simulink model "sim_BTMS"  (R2022b)
settings: Solver=FixedStepAuto  StartTime=0.0  StopTime=SimPara.t_sim  FixedStep=0.001  RelTol=1e-3
values from neighbouring files (symbols this model uses):
  BatPara = get_BatPara(BatPara, config_battery)    [sim_BTMS_interface.m]
  p = epe_mod(jj).p    [main_sim_BTMS_1_system_setup.m]
  SysPara = rmfield(SysPara, {'p','s'})    [main_sim_BTMS_1_system_setup.m]
undefined symbols (not defined in the file or in its folder): A, BTMSConfig, i, LSAPara, SimPara, x2_cal, x3_cal, x_cal
libraries: simulink x14, dspstat3 x7, dspindex x1
(part 4 of 4)

== system sim_BTMS/Monitoring and Logging/Load Spectrum Analysis/Load Spectrum Analysis ON/Load Spectrum Analysis ON/One parametric LSA of cell delta C-Rate/For Iterator val1 ==
  data_in : Inport
  data_in_delay : Inport  Port=2
  Add : Sum
  Assignment Subsystem : Subsystem  TreatAsAtomicUnit=on
  Constant : Constant  Value=bins_borders
  Constant2 : Constant
  Find Nonzero Elements : Find
  Iterate number of bins : ForIterator  ResetStates=reset  IterationLimit=length(bins_mean)  IterationVariableDataType=double
  Logical Operator : Logic  AllPortsSameDT=off  OutDataTypeStr=boolean
  Relational Operator : RelationalOperator  OutDataTypeStr=boolean  RndMeth=Simplest  InputSameDT=off
  Relational Operator1 : RelationalOperator  Operator=<  OutDataTypeStr=boolean  RndMeth=Simplest  InputSameDT=off
  select bin upper border : Selector  InputPortWidth=length(bins_borders)  IndexOptions=Index vector (port)  Indices=1:p  OutputSizes=1
  select parallel cell2 : Selector  InputPortWidth=length(bins_borders)  IndexOptions=Index vector (port)  Indices=1:p  OutputSizes=1
  LSA_out : Outport  VectorParamsAs1DForOutWhenUnconnected=off
  wires:
  data_in_delay/1 -> Assignment Subsystem/3(data_in_delayed)
  Constant/1 -> select bin upper border/1, select parallel cell2/1
  Add/1 -> select bin upper border/2
  Constant2/1 -> Add/1
  Iterate number of bins/1 -> Add/2, Assignment Subsystem/1(k), select parallel cell2/2
  select parallel cell2/1 -> Relational Operator/2
  select bin upper border/1 -> Relational Operator1/2
  data_in/1 -> Relational Operator1/1, Relational Operator/1
  Relational Operator1/1 -> Logical Operator/2
  Relational Operator/1 -> Logical Operator/1
  Logical Operator/1 -> Find Nonzero Elements/1
  Find Nonzero Elements/1 -> Assignment Subsystem/2(index_cell)
  Assignment Subsystem/1(LSA_out) -> LSA_out/1

== system sim_BTMS/Monitoring and Logging/Load Spectrum Analysis/Load Spectrum Analysis ON/Load Spectrum Analysis ON/One parametric LSA of cell delta temperature/For Iterator val1 ==
  data_in : Inport
  data_in_delay : Inport  Port=2
  Add : Sum
  Assignment Subsystem : Subsystem  TreatAsAtomicUnit=on
  Constant : Constant  Value=bins_borders
  Constant2 : Constant
  Find Nonzero Elements : Find
  Iterate number of bins : ForIterator  ResetStates=reset  IterationLimit=length(bins_mean)  IterationVariableDataType=double
  Logical Operator : Logic  AllPortsSameDT=off  OutDataTypeStr=boolean
  Relational Operator : RelationalOperator  OutDataTypeStr=boolean  RndMeth=Simplest  InputSameDT=off
  Relational Operator1 : RelationalOperator  Operator=<  OutDataTypeStr=boolean  RndMeth=Simplest  InputSameDT=off
  select bin upper border : Selector  InputPortWidth=length(bins_borders)  IndexOptions=Index vector (port)  Indices=1:p  OutputSizes=1
  select parallel cell2 : Selector  InputPortWidth=length(bins_borders)  IndexOptions=Index vector (port)  Indices=1:p  OutputSizes=1
  LSA_out : Outport  VectorParamsAs1DForOutWhenUnconnected=off
  wires:
  Assignment Subsystem/1(LSA_out) -> LSA_out/1
  Find Nonzero Elements/1 -> Assignment Subsystem/2(index_cell)
  Logical Operator/1 -> Find Nonzero Elements/1
  Relational Operator/1 -> Logical Operator/1
  Relational Operator1/1 -> Logical Operator/2
  data_in/1 -> Relational Operator/1, Relational Operator1/1
  select bin upper border/1 -> Relational Operator1/2
  select parallel cell2/1 -> Relational Operator/2
  Iterate number of bins/1 -> select parallel cell2/2, Assignment Subsystem/1(k), Add/2
  Constant2/1 -> Add/1
  Add/1 -> select bin upper border/2
  Constant/1 -> select parallel cell2/1, select bin upper border/1
  data_in_delay/1 -> Assignment Subsystem/3(data_in_delayed)

== system sim_BTMS/Monitoring and Logging/Load Spectrum Analysis/Load Spectrum Analysis ON/Load Spectrum Analysis ON/One parametric LSA of cell temperatures/For Iterator val1 ==
  data_in : Inport
  data_in_delay : Inport  Port=2
  Add : Sum
  Assignment Subsystem : Subsystem  TreatAsAtomicUnit=on
  Constant : Constant  Value=bins_borders
  Constant2 : Constant
  Find Nonzero Elements : Find
  Iterate number of bins : ForIterator  ResetStates=reset  IterationLimit=length(bins_mean)  IterationVariableDataType=double
  Logical Operator : Logic  AllPortsSameDT=off  OutDataTypeStr=boolean
  Relational Operator : RelationalOperator  OutDataTypeStr=boolean  RndMeth=Simplest  InputSameDT=off
  Relational Operator1 : RelationalOperator  Operator=<  OutDataTypeStr=boolean  RndMeth=Simplest  InputSameDT=off
  select bin upper border : Selector  InputPortWidth=length(bins_borders)  IndexOptions=Index vector (port)  Indices=1:p  OutputSizes=1
  select parallel cell2 : Selector  InputPortWidth=length(bins_borders)  IndexOptions=Index vector (port)  Indices=1:p  OutputSizes=1
  LSA_out : Outport  VectorParamsAs1DForOutWhenUnconnected=off
  wires:
  Assignment Subsystem/1(LSA_out) -> LSA_out/1
  Find Nonzero Elements/1 -> Assignment Subsystem/2(index_cell)
  Logical Operator/1 -> Find Nonzero Elements/1
  Relational Operator/1 -> Logical Operator/1
  Relational Operator1/1 -> Logical Operator/2
  data_in/1 -> Relational Operator/1, Relational Operator1/1
  select bin upper border/1 -> Relational Operator1/2
  select parallel cell2/1 -> Relational Operator/2
  Iterate number of bins/1 -> select parallel cell2/2, Assignment Subsystem/1(k), Add/2
  Constant2/1 -> Add/1
  Add/1 -> select bin upper border/2
  Constant/1 -> select parallel cell2/1, select bin upper border/1
  data_in_delay/1 -> Assignment Subsystem/3(data_in_delayed)

== system sim_BTMS/Monitoring and Logging/Load Spectrum Analysis/Load Spectrum Analysis ON/Load Spectrum Analysis ON/Subsystem1/SubsyMMatrssdatrixm ==
  In1 : Inport
  Enable : EnablePort  PropagateVarSize=During execution
  "summiert Dim. 4, die die Einzelzelle angibt" : Sum  Inputs=+  CollapseMode=Specified dimension  CollapseDim=dim
  Out1 : Outport  VectorParamsAs1DForOutWhenUnconnected=off
  wires:
  In1/1 -> "summiert Dim. 4, die die Einzelzelle angibt"/1
  "summiert Dim. 4, die die Einzelzelle angibt"/1 -> Out1/1

== system sim_BTMS/Monitoring and Logging/Load Spectrum Analysis/Load Spectrum Analysis ON/Load Spectrum Analysis ON/Subsystem2/SubsyMMatrssdatrixm ==
  In1 : Inport
  Enable : EnablePort  PropagateVarSize=During execution
  "summiert Dim. 4, die die Einzelzelle angibt" : Sum  Inputs=+  CollapseMode=Specified dimension  CollapseDim=dim
  Out1 : Outport  VectorParamsAs1DForOutWhenUnconnected=off
  wires:
  "summiert Dim. 4, die die Einzelzelle angibt"/1 -> Out1/1
  In1/1 -> "summiert Dim. 4, die die Einzelzelle angibt"/1

== system sim_BTMS/Monitoring and Logging/Load Spectrum Analysis/Load Spectrum Analysis ON/Load Spectrum Analysis ON/Subsystem3/SubsyMMatrssdatrixm ==
  In1 : Inport
  Enable : EnablePort  PropagateVarSize=During execution
  "summiert Dim. 4, die die Einzelzelle angibt" : Sum  Inputs=+  CollapseMode=Specified dimension  CollapseDim=dim
  Out1 : Outport  VectorParamsAs1DForOutWhenUnconnected=off
  wires:
  In1/1 -> "summiert Dim. 4, die die Einzelzelle angibt"/1
  "summiert Dim. 4, die die Einzelzelle angibt"/1 -> Out1/1

== system sim_BTMS/Monitoring and Logging/Load Spectrum Analysis/Load Spectrum Analysis ON/Load Spectrum Analysis ON/Subsystem4/SubsyMMatrssdatrixm ==
  In1 : Inport
  Enable : EnablePort  PropagateVarSize=During execution
  "summiert Dim. 4, die die Einzelzelle angibt" : Sum  Inputs=+  CollapseMode=Specified dimension  CollapseDim=dim
  Out1 : Outport  VectorParamsAs1DForOutWhenUnconnected=off
  wires:
  "summiert Dim. 4, die die Einzelzelle angibt"/1 -> Out1/1
  In1/1 -> "summiert Dim. 4, die die Einzelzelle angibt"/1

== system sim_BTMS/Monitoring and Logging/Load Spectrum Analysis/Load Spectrum Analysis ON/Load Spectrum Analysis ON/Subsystem5/SubsyMMatrssdatrixm ==
  In1 : Inport
  Enable : EnablePort  PropagateVarSize=During execution
  "summiert Dim. 4, die die Einzelzelle angibt" : Sum  Inputs=+  CollapseMode=Specified dimension  CollapseDim=dim
  Out1 : Outport  VectorParamsAs1DForOutWhenUnconnected=off
  wires:
  In1/1 -> "summiert Dim. 4, die die Einzelzelle angibt"/1
  "summiert Dim. 4, die die Einzelzelle angibt"/1 -> Out1/1

== system sim_BTMS/Monitoring and Logging/Load Spectrum Analysis/Load Spectrum Analysis ON/Load Spectrum Analysis ON/Subsystem6/SubsyMMatrssdatrixm ==
  In1 : Inport
  Enable : EnablePort  PropagateVarSize=During execution
  "summiert Dim. 4, die die Einzelzelle angibt" : Sum  Inputs=+  CollapseMode=Specified dimension  CollapseDim=dim
  Out1 : Outport  VectorParamsAs1DForOutWhenUnconnected=off
  wires:
  "summiert Dim. 4, die die Einzelzelle angibt"/1 -> Out1/1
  In1/1 -> "summiert Dim. 4, die die Einzelzelle angibt"/1

== system sim_BTMS/Monitoring and Logging/Load Spectrum Analysis/Load Spectrum Analysis ON/Load Spectrum Analysis ON/Subsystem7/SubsyMMatrssdatrixm ==
  In1 : Inport
  Enable : EnablePort  PropagateVarSize=During execution
  "summiert Dim. 4, die die Einzelzelle angibt" : Sum  Inputs=+  CollapseMode=Specified dimension  CollapseDim=dim
  Out1 : Outport  VectorParamsAs1DForOutWhenUnconnected=off
  wires:
  In1/1 -> "summiert Dim. 4, die die Einzelzelle angibt"/1
  "summiert Dim. 4, die die Einzelzelle angibt"/1 -> Out1/1

== system sim_BTMS/Monitoring and Logging/Load Spectrum Analysis/Load Spectrum Analysis ON/Load Spectrum Analysis ON/Subsystem8/SubsyMMatrssdatrixm ==
  In1 : Inport
  Enable : EnablePort  PropagateVarSize=During execution
  "summiert Dim. 4, die die Einzelzelle angibt" : Sum  Inputs=+  CollapseMode=Specified dimension  CollapseDim=dim
  Out1 : Outport  VectorParamsAs1DForOutWhenUnconnected=off
  wires:
  In1/1 -> "summiert Dim. 4, die die Einzelzelle angibt"/1
  "summiert Dim. 4, die die Einzelzelle angibt"/1 -> Out1/1

== system sim_BTMS/Monitoring and Logging/Load Spectrum Analysis/Load Spectrum Analysis ON/Load Spectrum Analysis ON/Subsystem9/SubsyMMatrssdatrixm ==
  In1 : Inport
  Enable : EnablePort  PropagateVarSize=During execution
  "summiert Dim. 4, die die Einzelzelle angibt" : Sum  Inputs=+  CollapseMode=Specified dimension  CollapseDim=dim
  Out1 : Outport  VectorParamsAs1DForOutWhenUnconnected=off
  wires:
  "summiert Dim. 4, die die Einzelzelle angibt"/1 -> Out1/1
  In1/1 -> "summiert Dim. 4, die die Einzelzelle angibt"/1

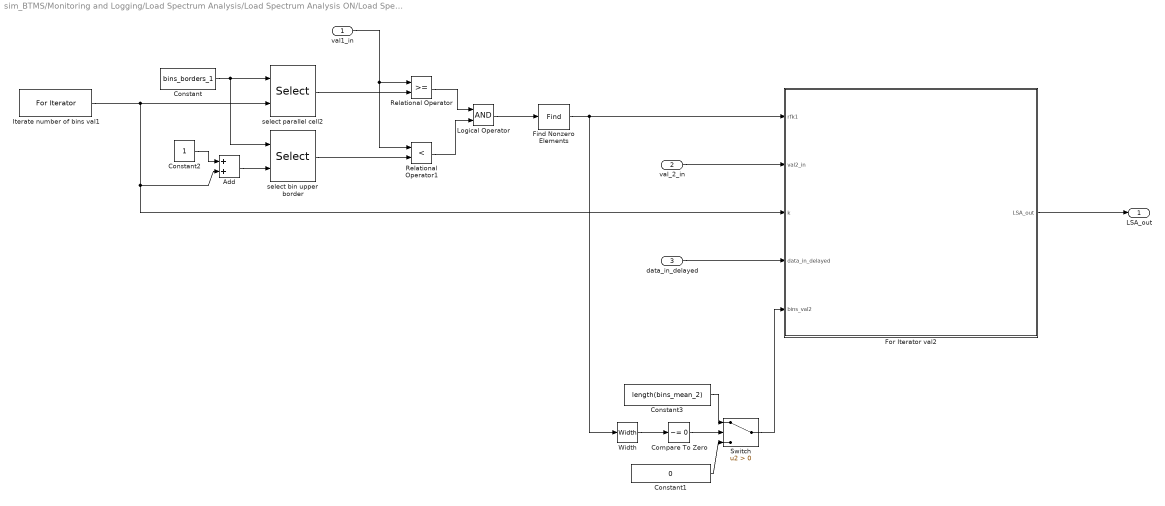
== system sim_BTMS/Monitoring and Logging/Load Spectrum Analysis/Load Spectrum Analysis ON/Load Spectrum Analysis ON/Two parametric LSA of cell C-Rate vs. temperature/For Iterator val1 ==
  val1_in : Inport
  val_2_in : Inport  Port=2
  data_in_delayed : Inport  Port=3
  Add : Sum
  Compare To Zero : simulink/Logic and Bit Operations/Compare To Zero  relop=~=  OutDataTypeStr=boolean
  Constant : Constant  Value=bins_borders_1
  Constant1 : Constant  Value=0
  Constant2 : Constant
  Constant3 : Constant  Value=length(bins_mean_2)
  Find Nonzero Elements : Find
  "For Iterator val2 " : Subsystem  TreatAsAtomicUnit=on
  Iterate number of bins val1 : ForIterator  ResetStates=reset  IterationLimit=length(bins_mean_1)  IterationVariableDataType=double
  Logical Operator : Logic  AllPortsSameDT=off  OutDataTypeStr=boolean
  Relational Operator : RelationalOperator  OutDataTypeStr=boolean  RndMeth=Simplest  InputSameDT=off
  Relational Operator1 : RelationalOperator  Operator=<  OutDataTypeStr=boolean  RndMeth=Simplest  InputSameDT=off
  Switch : Switch  Criteria=u2 > Threshold  SaturateOnIntegerOverflow=off  InputSameDT=off
  Width : Width
  select bin upper border : Selector  InputPortWidth=length(bins_borders_1)  IndexOptions=Index vector (port)  Indices=1:p  OutputSizes=1
  select parallel cell2 : Selector  InputPortWidth=length(bins_borders_1)  IndexOptions=Index vector (port)  Indices=1:p  OutputSizes=1
  LSA_out : Outport  VectorParamsAs1DForOutWhenUnconnected=off
  wires:
  val_2_in/1 -> "For Iterator val2 "/2(val2_in)
  Find Nonzero Elements/1 -> "For Iterator val2 "/1(rfk1), Width/1
  Logical Operator/1 -> Find Nonzero Elements/1
  Relational Operator/1 -> Logical Operator/1
  Relational Operator1/1 -> Logical Operator/2
  val1_in/1 -> Relational Operator/1, Relational Operator1/1
  select bin upper border/1 -> Relational Operator1/2
  select parallel cell2/1 -> Relational Operator/2
  Iterate number of bins val1/1 -> select parallel cell2/2, Add/2, "For Iterator val2 "/3(k)
  Constant2/1 -> Add/1
  Add/1 -> select bin upper border/2
  Constant/1 -> select parallel cell2/1, select bin upper border/1
  "For Iterator val2 "/1(LSA_out) -> LSA_out/1
  data_in_delayed/1 -> "For Iterator val2 "/4(data_in_delayed)
  Compare To Zero/1 -> Switch/2
  Constant1/1 -> Switch/3
  Width/1 -> Compare To Zero/1
  Switch/1 -> "For Iterator val2 "/5(bins_val2)
  Constant3/1 -> Switch/1

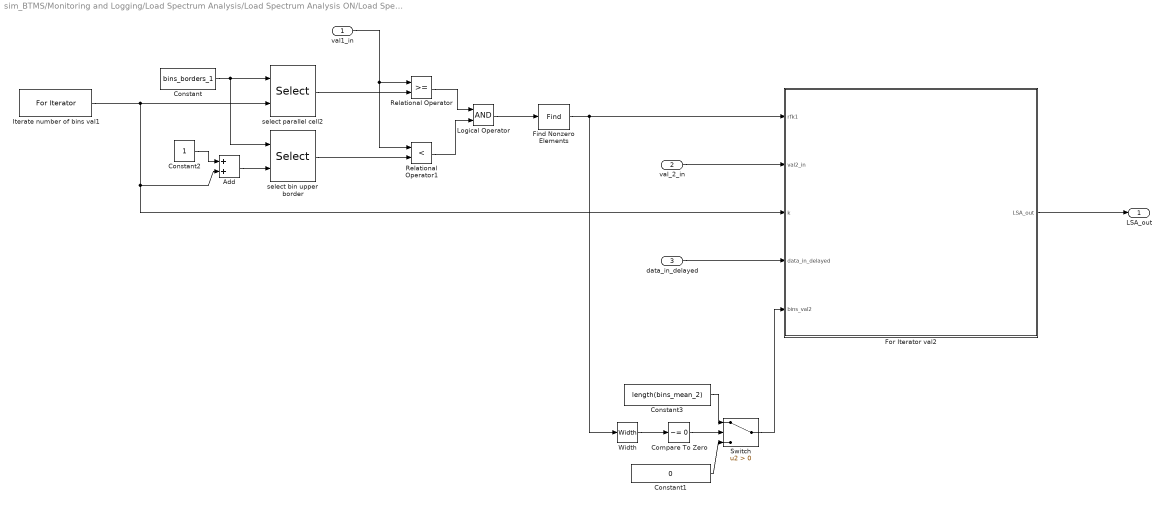
== system sim_BTMS/Monitoring and Logging/Load Spectrum Analysis/Load Spectrum Analysis ON/Load Spectrum Analysis ON/Two parametric LSA of cell SOC vs. C-Rate/For Iterator val1 ==
  val1_in : Inport
  val_2_in : Inport  Port=2
  data_in_delayed : Inport  Port=3
  Add : Sum
  Compare To Zero : simulink/Logic and Bit Operations/Compare To Zero  relop=~=  OutDataTypeStr=boolean
  Constant : Constant  Value=bins_borders_1
  Constant1 : Constant  Value=0
  Constant2 : Constant
  Constant3 : Constant  Value=length(bins_mean_2)
  Find Nonzero Elements : Find
  "For Iterator val2 " : Subsystem  TreatAsAtomicUnit=on
  Iterate number of bins val1 : ForIterator  ResetStates=reset  IterationLimit=length(bins_mean_1)  IterationVariableDataType=double
  Logical Operator : Logic  AllPortsSameDT=off  OutDataTypeStr=boolean
  Relational Operator : RelationalOperator  OutDataTypeStr=boolean  RndMeth=Simplest  InputSameDT=off
  Relational Operator1 : RelationalOperator  Operator=<  OutDataTypeStr=boolean  RndMeth=Simplest  InputSameDT=off
  Switch : Switch  Criteria=u2 > Threshold  SaturateOnIntegerOverflow=off  InputSameDT=off
  Width : Width
  select bin upper border : Selector  InputPortWidth=length(bins_borders_1)  IndexOptions=Index vector (port)  Indices=1:p  OutputSizes=1
  select parallel cell2 : Selector  InputPortWidth=length(bins_borders_1)  IndexOptions=Index vector (port)  Indices=1:p  OutputSizes=1
  LSA_out : Outport  VectorParamsAs1DForOutWhenUnconnected=off
  wires:
  Constant3/1 -> Switch/1
  Switch/1 -> "For Iterator val2 "/5(bins_val2)
  Width/1 -> Compare To Zero/1
  Constant1/1 -> Switch/3
  Compare To Zero/1 -> Switch/2
  data_in_delayed/1 -> "For Iterator val2 "/4(data_in_delayed)
  "For Iterator val2 "/1(LSA_out) -> LSA_out/1
  Constant/1 -> select bin upper border/1, select parallel cell2/1
  Add/1 -> select bin upper border/2
  Constant2/1 -> Add/1
  Iterate number of bins val1/1 -> "For Iterator val2 "/3(k), Add/2, select parallel cell2/2
  select parallel cell2/1 -> Relational Operator/2
  select bin upper border/1 -> Relational Operator1/2
  val1_in/1 -> Relational Operator1/1, Relational Operator/1
  Relational Operator1/1 -> Logical Operator/2
  Relational Operator/1 -> Logical Operator/1
  Logical Operator/1 -> Find Nonzero Elements/1
  Find Nonzero Elements/1 -> Width/1, "For Iterator val2 "/1(rfk1)
  val_2_in/1 -> "For Iterator val2 "/2(val2_in)

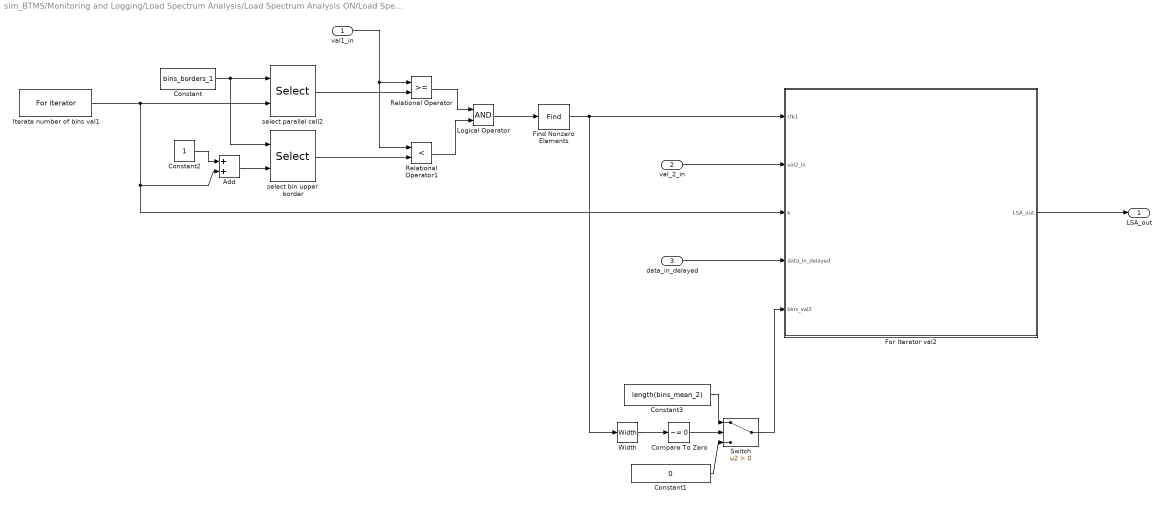
== system sim_BTMS/Monitoring and Logging/Load Spectrum Analysis/Load Spectrum Analysis ON/Load Spectrum Analysis ON/Two parametric LSA of cell SOC vs. temperature /For Iterator val1 ==
  val1_in : Inport
  val_2_in : Inport  Port=2
  data_in_delayed : Inport  Port=3
  Add : Sum
  Compare To Zero : simulink/Logic and Bit Operations/Compare To Zero  relop=~=  OutDataTypeStr=boolean
  Constant : Constant  Value=bins_borders_1
  Constant1 : Constant  Value=0
  Constant2 : Constant
  Constant3 : Constant  Value=length(bins_mean_2)
  Find Nonzero Elements : Find
  "For Iterator val2 " : Subsystem  TreatAsAtomicUnit=on
  Iterate number of bins val1 : ForIterator  ResetStates=reset  IterationLimit=length(bins_mean_1)  IterationVariableDataType=double
  Logical Operator : Logic  AllPortsSameDT=off  OutDataTypeStr=boolean
  Relational Operator : RelationalOperator  OutDataTypeStr=boolean  RndMeth=Simplest  InputSameDT=off
  Relational Operator1 : RelationalOperator  Operator=<  OutDataTypeStr=boolean  RndMeth=Simplest  InputSameDT=off
  Switch : Switch  Criteria=u2 > Threshold  SaturateOnIntegerOverflow=off  InputSameDT=off
  Width : Width
  select bin upper border : Selector  InputPortWidth=length(bins_borders_1)  IndexOptions=Index vector (port)  Indices=1:p  OutputSizes=1
  select parallel cell2 : Selector  InputPortWidth=length(bins_borders_1)  IndexOptions=Index vector (port)  Indices=1:p  OutputSizes=1
  LSA_out : Outport  VectorParamsAs1DForOutWhenUnconnected=off
  wires:
  Constant3/1 -> Switch/1
  Switch/1 -> "For Iterator val2 "/5(bins_val2)
  Width/1 -> Compare To Zero/1
  Constant1/1 -> Switch/3
  Compare To Zero/1 -> Switch/2
  data_in_delayed/1 -> "For Iterator val2 "/4(data_in_delayed)
  "For Iterator val2 "/1(LSA_out) -> LSA_out/1
  Constant/1 -> select bin upper border/1, select parallel cell2/1
  Add/1 -> select bin upper border/2
  Constant2/1 -> Add/1
  Iterate number of bins val1/1 -> "For Iterator val2 "/3(k), Add/2, select parallel cell2/2
  select parallel cell2/1 -> Relational Operator/2
  select bin upper border/1 -> Relational Operator1/2
  val1_in/1 -> Relational Operator1/1, Relational Operator/1
  Relational Operator1/1 -> Logical Operator/2
  Relational Operator/1 -> Logical Operator/1
  Logical Operator/1 -> Find Nonzero Elements/1
  Find Nonzero Elements/1 -> Width/1, "For Iterator val2 "/1(rfk1)
  val_2_in/1 -> "For Iterator val2 "/2(val2_in)

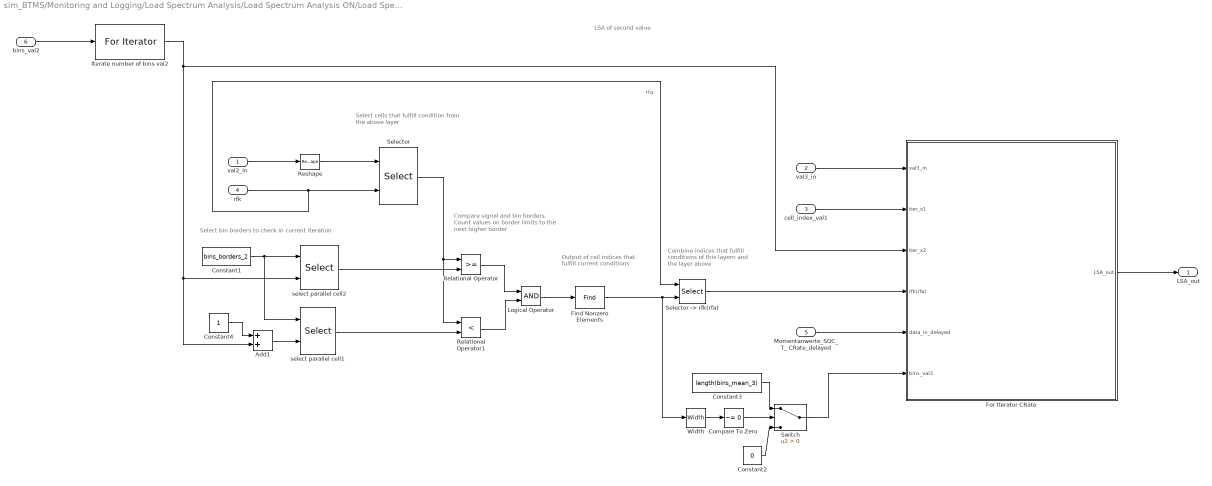
== system sim_BTMS/Monitoring and Logging/Load Spectrum Analysis/Load Spectrum Analysis ON/Load Spectrum Analysis ON/3-parametrische Momentanwertzählung SOC, T_Cells, CRate/For Iterator val1/For Iterator val2 ==
  note: Select cells that fulfill condition from the above layer
  note: LSA of second value
  note: rfa
  note: Select bin borders to check in current iteration
  note: Compare signal and bin borders. Count values on border limits to the next higher border
  note: Output of cell indices that fulfill current conditions
  note: Combine indices that fulfill conditions of this layern and the layer above
  val2_in : Inport
  val3_in : Inport  Port=2
  cell_index_val1 : Inport  Port=3
  rfk : Inport  Port=4
  Momentanwerte_SOC_T_ CRate_delayed : Inport  Port=5
  bins_val2 : Inport  Port=6
  Add1 : Sum
  Compare To Zero : simulink/Logic and Bit Operations/Compare To Zero  relop=~=  OutDataTypeStr=boolean
  Constant1 : Constant  Value=bins_borders_2
  Constant2 : Constant  Value=0
  Constant3 : Constant  Value=length(bins_mean_3)
  Constant4 : Constant
  Find Nonzero Elements : Find
  For Iterator CRate : Subsystem  TreatAsAtomicUnit=on
  Iterate number of bins val2 : ForIterator  ResetStates=reset  IterationSource=external  IterationLimit=length(x2_cal)  IterationVariableDataType=double
  Logical Operator : Logic  AllPortsSameDT=off  OutDataTypeStr=boolean
  Relational Operator : RelationalOperator  OutDataTypeStr=boolean  RndMeth=Simplest  InputSameDT=off
  Relational Operator1 : RelationalOperator  Operator=<  OutDataTypeStr=boolean  RndMeth=Simplest  InputSameDT=off
  Reshape : Reshape
  Selector : Selector  InputPortWidth=SysPara.p*SysPara.s  IndexOptions=Index vector (port)  Indices=1:p  OutputSizes=1
  "Selector -> rfk(rfa)" : Selector  InputPortWidth=SysPara.p*SysPara.s  IndexOptions=Index vector (port)  Indices=[1 3]  OutputSizes=1
  Switch : Switch  Criteria=u2 > Threshold  SaturateOnIntegerOverflow=off  InputSameDT=off
  Width : Width
  select parallel cell1 : Selector  InputPortWidth=length(bins_borders_2)  IndexOptions=Index vector (port)  Indices=1:p  OutputSizes=1
  select parallel cell2 : Selector  InputPortWidth=length(bins_borders_2)  IndexOptions=Index vector (port)  Indices=1:p  OutputSizes=1
  LSA_out : Outport  VectorParamsAs1DForOutWhenUnconnected=off
  wires:
  Switch/1 -> For Iterator CRate/6(bins_val3)
  Constant3/1 -> Switch/1
  Width/1 -> Compare To Zero/1
  Constant2/1 -> Switch/3
  Compare To Zero/1 -> Switch/2
  Find Nonzero Elements/1 -> "Selector -> rfk(rfa)"/2, Width/1
  bins_val2/1 -> Iterate number of bins val2/1
  val3_in/1 -> For Iterator CRate/1(val3_in)
  For Iterator CRate/1(LSA_out) -> LSA_out/1
  "Selector -> rfk(rfa)"/1 -> For Iterator CRate/4(rfk(rfa))
  rfk/1 -> Selector/2, "Selector -> rfk(rfa)"/1
  Logical Operator/1 -> Find Nonzero Elements/1
  Reshape/1 -> Selector/1
  val2_in/1 -> Reshape/1
  cell_index_val1/1 -> For Iterator CRate/2(iter_x1)
  Selector/1 -> Relational Operator/1, Relational Operator1/1
  Relational Operator/1 -> Logical Operator/1
  Relational Operator1/1 -> Logical Operator/2
  select parallel cell1/1 -> Relational Operator1/2
  select parallel cell2/1 -> Relational Operator/2
  Constant4/1 -> Add1/1
  Add1/1 -> select parallel cell1/2
  Iterate number of bins val2/1 -> select parallel cell2/2, Add1/2, For Iterator CRate/3(iter_x2)
  Constant1/1 -> select parallel cell2/1, select parallel cell1/1
  Momentanwerte_SOC_T_ CRate_delayed/1 -> For Iterator CRate/5(data_in_delayed)

== system sim_BTMS/Monitoring and Logging/Load Spectrum Analysis/Load Spectrum Analysis ON/Load Spectrum Analysis ON/One parametric LSA of cell C-Rate/For Iterator val1/Assignment Subsystem ==
  k : Inport
  index_cell : Inport  Port=2
  data_in_delayed : Inport  Port=3
  Add : Sum
  Assignment of matrix entries : Assignment  NumberOfDimensions=2  OutputInitialize=Specify size for each dimension in table  IndexOptions=Index vector (port),Index vector (port)  Indices=1,1  OutputSizes=length(bins_mean),SysPara.p*SysPara.s+1
  Constant1 : Constant  Value=SimPara.t_step
  "Selection of delayed matrix entries " : Selector  NumberOfDimensions=2  InputPortWidth=3  IndexOptions=Index vector (port),Index vector (port)  Indices=[1 3],1  OutputSizes=1,1
  LSA_out : Outport  VectorParamsAs1DForOutWhenUnconnected=off
  wires:
  index_cell/1 -> Assignment of matrix entries/3, "Selection of delayed matrix entries "/3
  Assignment of matrix entries/1 -> LSA_out/1
  k/1 -> "Selection of delayed matrix entries "/2, Assignment of matrix entries/2
  Constant1/1 -> Add/1
  "Selection of delayed matrix entries "/1 -> Add/2
  Add/1 -> Assignment of matrix entries/1
  data_in_delayed/1 -> "Selection of delayed matrix entries "/1

== system sim_BTMS/Monitoring and Logging/Load Spectrum Analysis/Load Spectrum Analysis ON/Load Spectrum Analysis ON/One parametric LSA of cell SOC/For Iterator val1/Assignment Subsystem ==
  k : Inport
  index_cell : Inport  Port=2
  data_in_delayed : Inport  Port=3
  Add : Sum
  Assignment of matrix entries : Assignment  NumberOfDimensions=2  OutputInitialize=Specify size for each dimension in table  IndexOptions=Index vector (port),Index vector (port)  Indices=1,1  OutputSizes=length(bins_mean),SysPara.p*SysPara.s+1
  Constant1 : Constant  Value=SimPara.t_step
  "Selection of delayed matrix entries " : Selector  NumberOfDimensions=2  InputPortWidth=3  IndexOptions=Index vector (port),Index vector (port)  Indices=[1 3],1  OutputSizes=1,1
  LSA_out : Outport  VectorParamsAs1DForOutWhenUnconnected=off
  wires:
  data_in_delayed/1 -> "Selection of delayed matrix entries "/1
  Add/1 -> Assignment of matrix entries/1
  "Selection of delayed matrix entries "/1 -> Add/2
  Constant1/1 -> Add/1
  k/1 -> Assignment of matrix entries/2, "Selection of delayed matrix entries "/2
  Assignment of matrix entries/1 -> LSA_out/1
  index_cell/1 -> "Selection of delayed matrix entries "/3, Assignment of matrix entries/3

== system sim_BTMS/Monitoring and Logging/Load Spectrum Analysis/Load Spectrum Analysis ON/Load Spectrum Analysis ON/One parametric LSA of cell delta C-Rate/For Iterator val1/Assignment Subsystem ==
  k : Inport
  index_cell : Inport  Port=2
  data_in_delayed : Inport  Port=3
  Add : Sum
  Assignment of matrix entries : Assignment  NumberOfDimensions=2  OutputInitialize=Specify size for each dimension in table  IndexOptions=Index vector (port),Index vector (port)  Indices=1,1  OutputSizes=length(bins_mean),SysPara.p*SysPara.s+1
  Constant1 : Constant  Value=SimPara.t_step
  "Selection of delayed matrix entries " : Selector  NumberOfDimensions=2  InputPortWidth=3  IndexOptions=Index vector (port),Index vector (port)  Indices=[1 3],1  OutputSizes=1,1
  LSA_out : Outport  VectorParamsAs1DForOutWhenUnconnected=off
  wires:
  data_in_delayed/1 -> "Selection of delayed matrix entries "/1
  Add/1 -> Assignment of matrix entries/1
  "Selection of delayed matrix entries "/1 -> Add/2
  Constant1/1 -> Add/1
  k/1 -> Assignment of matrix entries/2, "Selection of delayed matrix entries "/2
  Assignment of matrix entries/1 -> LSA_out/1
  index_cell/1 -> "Selection of delayed matrix entries "/3, Assignment of matrix entries/3

== system sim_BTMS/Monitoring and Logging/Load Spectrum Analysis/Load Spectrum Analysis ON/Load Spectrum Analysis ON/One parametric LSA of cell delta temperature/For Iterator val1/Assignment Subsystem ==
  k : Inport
  index_cell : Inport  Port=2
  data_in_delayed : Inport  Port=3
  Add : Sum
  Assignment of matrix entries : Assignment  NumberOfDimensions=2  OutputInitialize=Specify size for each dimension in table  IndexOptions=Index vector (port),Index vector (port)  Indices=1,1  OutputSizes=length(bins_mean),SysPara.p*SysPara.s+1
  Constant1 : Constant  Value=SimPara.t_step
  "Selection of delayed matrix entries " : Selector  NumberOfDimensions=2  InputPortWidth=3  IndexOptions=Index vector (port),Index vector (port)  Indices=[1 3],1  OutputSizes=1,1
  LSA_out : Outport  VectorParamsAs1DForOutWhenUnconnected=off
  wires:
  index_cell/1 -> Assignment of matrix entries/3, "Selection of delayed matrix entries "/3
  Assignment of matrix entries/1 -> LSA_out/1
  k/1 -> "Selection of delayed matrix entries "/2, Assignment of matrix entries/2
  Constant1/1 -> Add/1
  "Selection of delayed matrix entries "/1 -> Add/2
  Add/1 -> Assignment of matrix entries/1
  data_in_delayed/1 -> "Selection of delayed matrix entries "/1

== system sim_BTMS/Monitoring and Logging/Load Spectrum Analysis/Load Spectrum Analysis ON/Load Spectrum Analysis ON/One parametric LSA of cell temperatures/For Iterator val1/Assignment Subsystem ==
  k : Inport
  index_cell : Inport  Port=2
  data_in_delayed : Inport  Port=3
  Add : Sum
  Assignment of matrix entries : Assignment  NumberOfDimensions=2  OutputInitialize=Specify size for each dimension in table  IndexOptions=Index vector (port),Index vector (port)  Indices=1,1  OutputSizes=length(bins_mean),SysPara.p*SysPara.s+1
  Constant1 : Constant  Value=SimPara.t_step
  "Selection of delayed matrix entries " : Selector  NumberOfDimensions=2  InputPortWidth=3  IndexOptions=Index vector (port),Index vector (port)  Indices=[1 3],1  OutputSizes=1,1
  LSA_out : Outport  VectorParamsAs1DForOutWhenUnconnected=off
  wires:
  index_cell/1 -> Assignment of matrix entries/3, "Selection of delayed matrix entries "/3
  Assignment of matrix entries/1 -> LSA_out/1
  k/1 -> "Selection of delayed matrix entries "/2, Assignment of matrix entries/2
  Constant1/1 -> Add/1
  "Selection of delayed matrix entries "/1 -> Add/2
  Add/1 -> Assignment of matrix entries/1
  data_in_delayed/1 -> "Selection of delayed matrix entries "/1

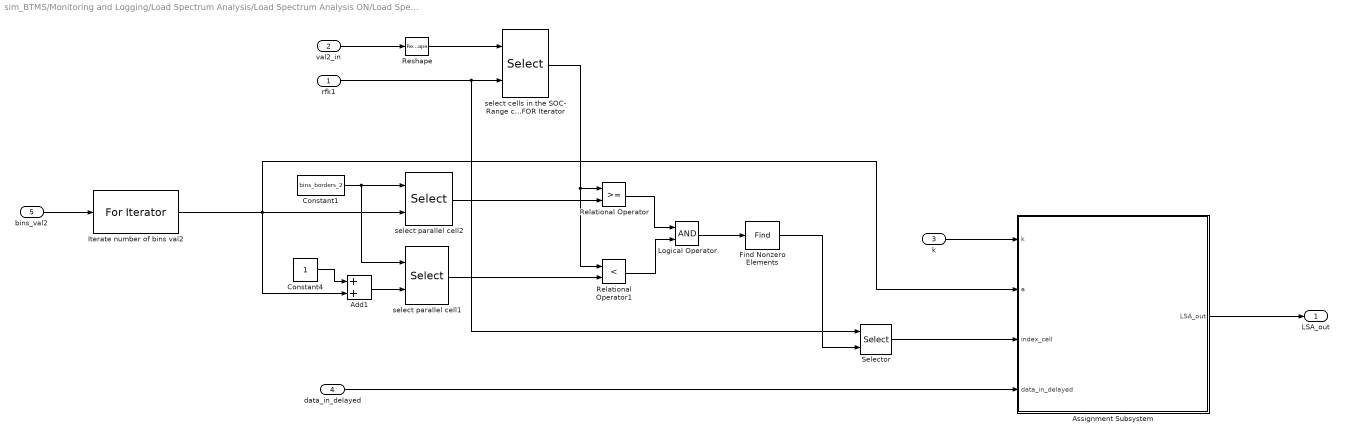
== system sim_BTMS/Monitoring and Logging/Load Spectrum Analysis/Load Spectrum Analysis ON/Load Spectrum Analysis ON/Two parametric LSA of cell C-Rate vs. temperature/For Iterator val1/For Iterator val2  ==
  rfk1 : Inport
  val2_in : Inport  Port=2
  k : Inport  Port=3
  data_in_delayed : Inport  Port=4
  bins_val2 : Inport  Port=5
  Add1 : Sum
  Assignment Subsystem : Subsystem  TreatAsAtomicUnit=on
  Constant1 : Constant  Value=bins_borders_2
  Constant4 : Constant
  Find Nonzero Elements : Find
  Iterate number of bins val2 : ForIterator  ResetStates=reset  IterationSource=external  IterationLimit=length(x_cal)  IterationVariableDataType=double
  Logical Operator : Logic  AllPortsSameDT=off  OutDataTypeStr=boolean
  Relational Operator : RelationalOperator  OutDataTypeStr=boolean  RndMeth=Simplest  InputSameDT=off
  Relational Operator1 : RelationalOperator  Operator=<  OutDataTypeStr=boolean  RndMeth=Simplest  InputSameDT=off
  Reshape : Reshape
  Selector : Selector  InputPortWidth=SysPara.p*SysPara.s  IndexOptions=Index vector (port)  Indices=[1 3]  OutputSizes=1
  select cells in the SOC- Range corresponding to 1. FOR Iterator : Selector  InputPortWidth=SysPara.p*SysPara.s  IndexOptions=Index vector (port)  Indices=1:p  OutputSizes=1
  select parallel cell1 : Selector  InputPortWidth=length(bins_borders_2)  IndexOptions=Index vector (port)  Indices=1:p  OutputSizes=1
  select parallel cell2 : Selector  InputPortWidth=length(bins_borders_2)  IndexOptions=Index vector (port)  Indices=1:p  OutputSizes=1
  LSA_out : Outport  VectorParamsAs1DForOutWhenUnconnected=off
  wires:
  Assignment Subsystem/1(LSA_out) -> LSA_out/1
  Selector/1 -> Assignment Subsystem/3(index_cell)
  Find Nonzero Elements/1 -> Selector/2
  rfk1/1 -> select cells in the SOC- Range corresponding to 1. FOR Iterator/2, Selector/1
  Logical Operator/1 -> Find Nonzero Elements/1
  Reshape/1 -> select cells in the SOC- Range corresponding to 1. FOR Iterator/1
  val2_in/1 -> Reshape/1
  k/1 -> Assignment Subsystem/1(k)
  select cells in the SOC- Range corresponding to 1. FOR Iterator/1 -> Relational Operator/1, Relational Operator1/1
  Relational Operator/1 -> Logical Operator/1
  Relational Operator1/1 -> Logical Operator/2
  select parallel cell1/1 -> Relational Operator1/2
  select parallel cell2/1 -> Relational Operator/2
  Constant4/1 -> Add1/1
  Add1/1 -> select parallel cell1/2
  Iterate number of bins val2/1 -> Add1/2, Assignment Subsystem/2(a), select parallel cell2/2
  Constant1/1 -> select parallel cell2/1, select parallel cell1/1
  data_in_delayed/1 -> Assignment Subsystem/4(data_in_delayed)
  bins_val2/1 -> Iterate number of bins val2/1

== system sim_BTMS/Monitoring and Logging/Load Spectrum Analysis/Load Spectrum Analysis ON/Load Spectrum Analysis ON/Two parametric LSA of cell SOC vs. C-Rate/For Iterator val1/For Iterator val2  ==
  rfk1 : Inport
  val2_in : Inport  Port=2
  k : Inport  Port=3
  data_in_delayed : Inport  Port=4
  bins_val2 : Inport  Port=5
  Add1 : Sum
  Assignment Subsystem : Subsystem  TreatAsAtomicUnit=on
  Constant1 : Constant  Value=bins_borders_2
  Constant4 : Constant
  Find Nonzero Elements : Find
  Iterate number of bins val2 : ForIterator  ResetStates=reset  IterationSource=external  IterationLimit=length(x_cal)  IterationVariableDataType=double
  Logical Operator : Logic  AllPortsSameDT=off  OutDataTypeStr=boolean
  Relational Operator : RelationalOperator  OutDataTypeStr=boolean  RndMeth=Simplest  InputSameDT=off
  Relational Operator1 : RelationalOperator  Operator=<  OutDataTypeStr=boolean  RndMeth=Simplest  InputSameDT=off
  Reshape : Reshape
  Selector : Selector  InputPortWidth=SysPara.p*SysPara.s  IndexOptions=Index vector (port)  Indices=[1 3]  OutputSizes=1
  select cells in the SOC- Range corresponding to 1. FOR Iterator : Selector  InputPortWidth=SysPara.p*SysPara.s  IndexOptions=Index vector (port)  Indices=1:p  OutputSizes=1
  select parallel cell1 : Selector  InputPortWidth=length(bins_borders_2)  IndexOptions=Index vector (port)  Indices=1:p  OutputSizes=1
  select parallel cell2 : Selector  InputPortWidth=length(bins_borders_2)  IndexOptions=Index vector (port)  Indices=1:p  OutputSizes=1
  LSA_out : Outport  VectorParamsAs1DForOutWhenUnconnected=off
  wires:
  bins_val2/1 -> Iterate number of bins val2/1
  data_in_delayed/1 -> Assignment Subsystem/4(data_in_delayed)
  Constant1/1 -> select parallel cell1/1, select parallel cell2/1
  Iterate number of bins val2/1 -> select parallel cell2/2, Assignment Subsystem/2(a), Add1/2
  Add1/1 -> select parallel cell1/2
  Constant4/1 -> Add1/1
  select parallel cell2/1 -> Relational Operator/2
  select parallel cell1/1 -> Relational Operator1/2
  Relational Operator1/1 -> Logical Operator/2
  Relational Operator/1 -> Logical Operator/1
  select cells in the SOC- Range corresponding to 1. FOR Iterator/1 -> Relational Operator1/1, Relational Operator/1
  k/1 -> Assignment Subsystem/1(k)
  val2_in/1 -> Reshape/1
  Reshape/1 -> select cells in the SOC- Range corresponding to 1. FOR Iterator/1
  Logical Operator/1 -> Find Nonzero Elements/1
  rfk1/1 -> Selector/1, select cells in the SOC- Range corresponding to 1. FOR Iterator/2
  Find Nonzero Elements/1 -> Selector/2
  Selector/1 -> Assignment Subsystem/3(index_cell)
  Assignment Subsystem/1(LSA_out) -> LSA_out/1

== system sim_BTMS/Monitoring and Logging/Load Spectrum Analysis/Load Spectrum Analysis ON/Load Spectrum Analysis ON/Two parametric LSA of cell SOC vs. temperature /For Iterator val1/For Iterator val2  ==
  rfk1 : Inport
  val2_in : Inport  Port=2
  k : Inport  Port=3
  data_in_delayed : Inport  Port=4
  bins_val2 : Inport  Port=5
  Add1 : Sum
  Assignment Subsystem : Subsystem  TreatAsAtomicUnit=on
  Constant1 : Constant  Value=bins_borders_2
  Constant4 : Constant
  Find Nonzero Elements : Find
  Iterate number of bins val2 : ForIterator  ResetStates=reset  IterationSource=external  IterationLimit=length(x_cal)  IterationVariableDataType=double
  Logical Operator : Logic  AllPortsSameDT=off  OutDataTypeStr=boolean
  Relational Operator : RelationalOperator  OutDataTypeStr=boolean  RndMeth=Simplest  InputSameDT=off
  Relational Operator1 : RelationalOperator  Operator=<  OutDataTypeStr=boolean  RndMeth=Simplest  InputSameDT=off
  Reshape : Reshape
  Selector : Selector  InputPortWidth=SysPara.p*SysPara.s  IndexOptions=Index vector (port)  Indices=[1 3]  OutputSizes=1
  select cells in the SOC- Range corresponding to 1. FOR Iterator : Selector  InputPortWidth=SysPara.p*SysPara.s  IndexOptions=Index vector (port)  Indices=1:p  OutputSizes=1
  select parallel cell1 : Selector  InputPortWidth=length(bins_borders_2)  IndexOptions=Index vector (port)  Indices=1:p  OutputSizes=1
  select parallel cell2 : Selector  InputPortWidth=length(bins_borders_2)  IndexOptions=Index vector (port)  Indices=1:p  OutputSizes=1
  LSA_out : Outport  VectorParamsAs1DForOutWhenUnconnected=off
  wires:
  bins_val2/1 -> Iterate number of bins val2/1
  data_in_delayed/1 -> Assignment Subsystem/4(data_in_delayed)
  Constant1/1 -> select parallel cell1/1, select parallel cell2/1
  Iterate number of bins val2/1 -> select parallel cell2/2, Assignment Subsystem/2(a), Add1/2
  Add1/1 -> select parallel cell1/2
  Constant4/1 -> Add1/1
  select parallel cell2/1 -> Relational Operator/2
  select parallel cell1/1 -> Relational Operator1/2
  Relational Operator1/1 -> Logical Operator/2
  Relational Operator/1 -> Logical Operator/1
  select cells in the SOC- Range corresponding to 1. FOR Iterator/1 -> Relational Operator1/1, Relational Operator/1
  k/1 -> Assignment Subsystem/1(k)
  val2_in/1 -> Reshape/1
  Reshape/1 -> select cells in the SOC- Range corresponding to 1. FOR Iterator/1
  Logical Operator/1 -> Find Nonzero Elements/1
  rfk1/1 -> Selector/1, select cells in the SOC- Range corresponding to 1. FOR Iterator/2
  Find Nonzero Elements/1 -> Selector/2
  Selector/1 -> Assignment Subsystem/3(index_cell)
  Assignment Subsystem/1(LSA_out) -> LSA_out/1

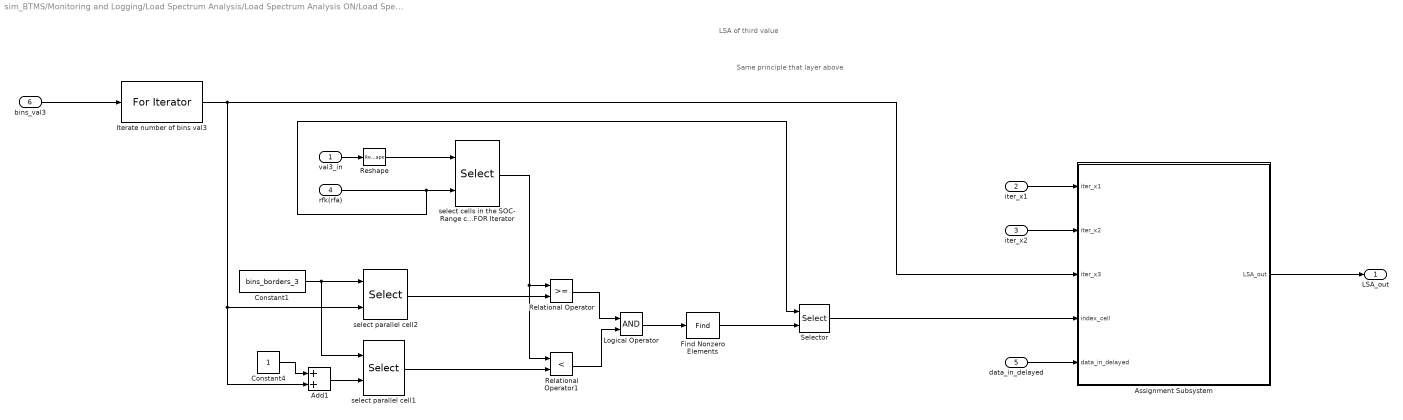
== system sim_BTMS/Monitoring and Logging/Load Spectrum Analysis/Load Spectrum Analysis ON/Load Spectrum Analysis ON/3-parametrische Momentanwertzählung SOC, T_Cells, CRate/For Iterator val1/For Iterator val2/For Iterator CRate ==
  note: Same principle that layer above
  note: LSA of third value
  val3_in : Inport
  iter_x1 : Inport  Port=2
  iter_x2 : Inport  Port=3
  rfk(rfa) : Inport  Port=4
  data_in_delayed : Inport  Port=5
  bins_val3 : Inport  Port=6
  Add1 : Sum
  Assignment Subsystem : Subsystem  TreatAsAtomicUnit=on
  Constant1 : Constant  Value=bins_borders_3
  Constant4 : Constant
  Find Nonzero Elements : Find
  Iterate number of bins val3 : ForIterator  ResetStates=reset  IterationSource=external  IterationLimit=length(x3_cal)  IterationVariableDataType=double
  Logical Operator : Logic  AllPortsSameDT=off  OutDataTypeStr=boolean
  Relational Operator : RelationalOperator  OutDataTypeStr=boolean  RndMeth=Simplest  InputSameDT=off
  Relational Operator1 : RelationalOperator  Operator=<  OutDataTypeStr=boolean  RndMeth=Simplest  InputSameDT=off
  Reshape : Reshape
  Selector : Selector  InputPortWidth=SysPara.p*SysPara.s  IndexOptions=Index vector (port)  Indices=[1 3]  OutputSizes=1
  select cells in the SOC- Range corresponding to 1. FOR Iterator : Selector  InputPortWidth=SysPara.p*SysPara.s  IndexOptions=Index vector (port)  Indices=1:p  OutputSizes=1
  select parallel cell1 : Selector  InputPortWidth=length(bins_borders_3)  IndexOptions=Index vector (port)  Indices=1:p  OutputSizes=1
  select parallel cell2 : Selector  InputPortWidth=length(bins_borders_3)  IndexOptions=Index vector (port)  Indices=1:p  OutputSizes=1
  LSA_out : Outport  VectorParamsAs1DForOutWhenUnconnected=off
  wires:
  Find Nonzero Elements/1 -> Selector/2
  bins_val3/1 -> Iterate number of bins val3/1
  rfk(rfa)/1 -> select cells in the SOC- Range corresponding to 1. FOR Iterator/2, Selector/1
  Logical Operator/1 -> Find Nonzero Elements/1
  Reshape/1 -> select cells in the SOC- Range corresponding to 1. FOR Iterator/1
  val3_in/1 -> Reshape/1
  select cells in the SOC- Range corresponding to 1. FOR Iterator/1 -> Relational Operator/1, Relational Operator1/1
  Relational Operator/1 -> Logical Operator/1
  Relational Operator1/1 -> Logical Operator/2
  select parallel cell1/1 -> Relational Operator1/2
  select parallel cell2/1 -> Relational Operator/2
  Constant4/1 -> Add1/1
  Add1/1 -> select parallel cell1/2
  Iterate number of bins val3/1 -> select parallel cell2/2, Add1/2, Assignment Subsystem/3(iter_x3)
  Constant1/1 -> select parallel cell2/1, select parallel cell1/1
  iter_x2/1 -> Assignment Subsystem/2(iter_x2)
  Assignment Subsystem/1(LSA_out) -> LSA_out/1
  iter_x1/1 -> Assignment Subsystem/1(iter_x1)
  data_in_delayed/1 -> Assignment Subsystem/5(data_in_delayed)
  Selector/1 -> Assignment Subsystem/4(index_cell)

== system sim_BTMS/Monitoring and Logging/Load Spectrum Analysis/Load Spectrum Analysis ON/Load Spectrum Analysis ON/Two parametric LSA of cell C-Rate vs. temperature/For Iterator val1/For Iterator val2 /Assignment Subsystem ==
  k : Inport
  a : Inport  Port=2
  index_cell : Inport  Port=3
  data_in_delayed : Inport  Port=4
  Add : Sum
  Assignment of matrix entries : Assignment  NumberOfDimensions=3  OutputInitialize=Specify size for each dimension in table  IndexOptions=Index vector (port),Index vector (port),Index vector (port)  Indices=1,1,1  OutputSizes=length(bins_mean_1),length(bins_mean_2),SysPara.p*SysPara.s+1
  Constant1 : Constant  Value=SimPara.t_step
  "Selection of delayed matrix entries " : Selector  NumberOfDimensions=3  InputPortWidth=3  IndexOptions=Index vector (port),Index vector (port),Index vector (port)  Indices=[1 3],1,1  OutputSizes=1,1,1
  LSA_out : Outport  VectorParamsAs1DForOutWhenUnconnected=off
  wires:
  index_cell/1 -> "Selection of delayed matrix entries "/4, Assignment of matrix entries/4
  Assignment of matrix entries/1 -> LSA_out/1
  a/1 -> Assignment of matrix entries/3, "Selection of delayed matrix entries "/3
  k/1 -> Assignment of matrix entries/2, "Selection of delayed matrix entries "/2
  Constant1/1 -> Add/1
  "Selection of delayed matrix entries "/1 -> Add/2
  Add/1 -> Assignment of matrix entries/1
  data_in_delayed/1 -> "Selection of delayed matrix entries "/1

== system sim_BTMS/Monitoring and Logging/Load Spectrum Analysis/Load Spectrum Analysis ON/Load Spectrum Analysis ON/Two parametric LSA of cell SOC vs. C-Rate/For Iterator val1/For Iterator val2 /Assignment Subsystem ==
  k : Inport
  a : Inport  Port=2
  index_cell : Inport  Port=3
  data_in_delayed : Inport  Port=4
  Add : Sum
  Assignment of matrix entries : Assignment  NumberOfDimensions=3  OutputInitialize=Specify size for each dimension in table  IndexOptions=Index vector (port),Index vector (port),Index vector (port)  Indices=1,1,1  OutputSizes=length(bins_mean_1),length(bins_mean_2),SysPara.p*SysPara.s+1
  Constant1 : Constant  Value=SimPara.t_step
  "Selection of delayed matrix entries " : Selector  NumberOfDimensions=3  InputPortWidth=3  IndexOptions=Index vector (port),Index vector (port),Index vector (port)  Indices=[1 3],1,1  OutputSizes=1,1,1
  LSA_out : Outport  VectorParamsAs1DForOutWhenUnconnected=off
  wires:
  data_in_delayed/1 -> "Selection of delayed matrix entries "/1
  Add/1 -> Assignment of matrix entries/1
  "Selection of delayed matrix entries "/1 -> Add/2
  Constant1/1 -> Add/1
  k/1 -> "Selection of delayed matrix entries "/2, Assignment of matrix entries/2
  a/1 -> "Selection of delayed matrix entries "/3, Assignment of matrix entries/3
  Assignment of matrix entries/1 -> LSA_out/1
  index_cell/1 -> Assignment of matrix entries/4, "Selection of delayed matrix entries "/4

== system sim_BTMS/Monitoring and Logging/Load Spectrum Analysis/Load Spectrum Analysis ON/Load Spectrum Analysis ON/Two parametric LSA of cell SOC vs. temperature /For Iterator val1/For Iterator val2 /Assignment Subsystem ==
  k : Inport
  a : Inport  Port=2
  index_cell : Inport  Port=3
  data_in_delayed : Inport  Port=4
  Add : Sum
  Assignment of matrix entries : Assignment  NumberOfDimensions=3  OutputInitialize=Specify size for each dimension in table  IndexOptions=Index vector (port),Index vector (port),Index vector (port)  Indices=1,1,1  OutputSizes=length(bins_mean_1),length(bins_mean_2),SysPara.p*SysPara.s+1
  Constant1 : Constant  Value=SimPara.t_step
  "Selection of delayed matrix entries " : Selector  NumberOfDimensions=3  InputPortWidth=3  IndexOptions=Index vector (port),Index vector (port),Index vector (port)  Indices=[1 3],1,1  OutputSizes=1,1,1
  LSA_out : Outport  VectorParamsAs1DForOutWhenUnconnected=off
  wires:
  data_in_delayed/1 -> "Selection of delayed matrix entries "/1
  Add/1 -> Assignment of matrix entries/1
  "Selection of delayed matrix entries "/1 -> Add/2
  Constant1/1 -> Add/1
  k/1 -> "Selection of delayed matrix entries "/2, Assignment of matrix entries/2
  a/1 -> "Selection of delayed matrix entries "/3, Assignment of matrix entries/3
  Assignment of matrix entries/1 -> LSA_out/1
  index_cell/1 -> Assignment of matrix entries/4, "Selection of delayed matrix entries "/4

== system sim_BTMS/Monitoring and Logging/Load Spectrum Analysis/Load Spectrum Analysis ON/Load Spectrum Analysis ON/3-parametrische Momentanwertzählung SOC, T_Cells, CRate/For Iterator val1/For Iterator val2/For Iterator CRate/Assignment Subsystem ==
  note: Assign updated value to tensor of last time-step
  note: Select field that will get updated in this time-step
  iter_x1 : Inport
  iter_x2 : Inport  Port=2
  iter_x3 : Inport  Port=3
  index_cell : Inport  Port=4
  data_in_delayed : Inport  Port=5
  Add : Sum
  Assignment of matrix entries : Assignment  NumberOfDimensions=4  OutputInitialize=Specify size for each dimension in table  IndexOptions=Index vector (port),Index vector (port),Index vector (port),Index vector (port)  Indices=1,1,1,1  OutputSizes=length(bins_mean_1),length(bins_mean_2),length(bins_mean_3),SysPara.p*SysPara.s+1
  Constant1 : Constant  Value=SimPara.t_step
  "Selection of delayed matrix entries " : Selector  NumberOfDimensions=4  InputPortWidth=3  IndexOptions=Index vector (port),Index vector (port),Index vector (port),Index vector (port)  Indices=[1 3],1,1,1  OutputSizes=1,1,1,1
  LSA_out : Outport  VectorParamsAs1DForOutWhenUnconnected=off
  wires:
  iter_x3/1 -> Assignment of matrix entries/4, "Selection of delayed matrix entries "/4
  index_cell/1 -> "Selection of delayed matrix entries "/5, Assignment of matrix entries/5
  Assignment of matrix entries/1 -> LSA_out/1
  iter_x2/1 -> Assignment of matrix entries/3, "Selection of delayed matrix entries "/3
  iter_x1/1 -> Assignment of matrix entries/2, "Selection of delayed matrix entries "/2
  Constant1/1 -> Add/1
  "Selection of delayed matrix entries "/1 -> Add/2
  Add/1 -> Assignment of matrix entries/1
  data_in_delayed/1 -> "Selection of delayed matrix entries "/1

== matlab function sim_BTMS/Create BTMS input/BTMS fluid simulation/BTMS fluid simulation function ==
  data: T_cell input size=[SysPara.p, SysPara.s]; T_fluid_BTMS input; Vdot_BTMS input; BTMSConfig parameter; max_T_channel_out output size=1; T_cell_ambient output size=[SysPara.p, SysPara.s]; alpha_cell_ambient output size=[SysPara.p, SysPara.s]; A_x input; A_y input; A_z input; s input; p input; BatPara parameter
function [max_T_channel_out, T_cell_ambient, alpha_cell_ambient] = create_BTMS_input(T_cell, T_fluid_BTMS, Vdot_BTMS, BTMSConfig, A_x, A_y, A_z, s, p, BatPara)

%% Inputs

% T_cell          Cell temperature matrix in °C
% T_fluid_BTMS    Inlet temperature of cooling fluid in °C
% Vdot_BTMS       Overall fluid mass flow in m^3/s (needed for dynamic adaption of heat transfer coefficients. Currently unused.)


%% Transform T_cell to column vector

T_cell_vec = reshape(T_cell, [numel(T_cell),1]);


%% Some necessary variables

A_dir = [A_x, A_y, A_z];
A_cell_total = BatPara.physical.A;


%% Get average temperature of cells adjacent to the cooling channels

T_avg_cell_channel = NaN(BTMSConfig.num_channels, 1);
for ii = 1:BTMSConfig.num_channels
    T_avg_cell_channel(ii) = sum(T_cell_vec(nonzeros(BTMSConfig.channel_def_mat(ii,:))'))/BTMSConfig.channel_num_adj_cells(ii);
end


%% Get volume and mass flow and speed through each cooling channel

% Done once outside of simulation in 'create_BTMS_config.m'
% For the model to support dynamic Vdot_BTMS inlet temperatures copy the
% code into this function!


%% Calculate channel heat transfer coefficient

% Done once outside of simulation in 'create_BTMS_config.m'
% For the model to support dynamic Vdot_BTMS inlet temperatures copy the
% code into this function!


%% Calculate average cooling channel temp

T_channel_out = NaN(BTMSConfig.num_channels, 1);
for ii = 1:BTMSConfig.num_channels
    T_channel_out(ii) = get_fluid_out_temp(T_fluid_BTMS, T_avg_cell_channel(ii), BTMSConfig.channel_length(ii), BTMSConfig.channel_mdot(ii), BTMSConfig.fluid_para.cp, BTMSConfig.lambda_wall);
end

T_channel_avg = (T_fluid_BTMS + T_channel_out) / 2;



%% Write values is vectors

% T_cell_ambient_vec: Meat temperature around each cell
% alpha_cell_ambient_vec: Scaled heat transfer coefficient

[alpha_cell_ambient_vec, T_cell_ambient_vec]  = cal_output_vecs(T_channel_avg, BTMSConfig.channel_alpha, BTMSConfig.channel_def_mat, BTMSConfig.channel_orientation, A_dir, A_cell_total, s * p);



%% Recreate matrix structure for sim_battery_system

T_cell_ambient = reshape(T_cell_ambient_vec, [p, s]);
alpha_cell_ambient = reshape(alpha_cell_ambient_vec, [p, s]);

max_T_channel_out = max(T_channel_out);


end

function T_channel_out = get_fluid_out_temp(T_channel_in, T_avg_cell, channel_length, mdot, c_p_fluid, lambda_wall)
% Calculate approximated channel output temperature
% Approximation for axial flow in pipe

epsilon = lambda_wall / (mdot * c_p_fluid);
T_channel_out = (T_channel_in - T_avg_cell) * exp(-epsilon*channel_length) + T_avg_cell;  
    
end


function [alpha_cell_ambient_vec, T_cell_ambient_vec]  = cal_output_vecs(T_channel_avg, alpha_channel, channel_def_mat, channel_orientation, A_dir, A_cell_total, number_of_cells)

% Preallocate output vectors
alpha_cell_ambient_vec = zeros(1, number_of_cells);
T_cell_ambient_vec = zeros(1, number_of_cells);

for ii = 1:number_of_cells
    
    % Look if a cell is adjacent to one or more cooling channels
    [row, ~] = find(channel_def_mat == ii);
        if length(row) >= 1     % Cell is in contact with one or more cooling channels
            
            % Calculate mean temperature around cell
            T_cell_ambient_vec(ii) = sum(T_channel_avg(row)) / length(row);
            
            % Get vector with area of heat transfers
            A_heat_total_cell = zeros(length(row), 1);
            
            x_dir = find(channel_orientation(row) == 'x');
            y_dir = find(channel_orientation(row) == 'y');
            z_dir = find(channel_orientation(row) == 'z');
            
            A_heat_total_cell(x_dir) = A_dir(1);
            A_heat_total_cell(y_dir) = A_dir(2);
            A_heat_total_cell(z_dir) = A_dir(3);
            
            % Calculate scaled heat transfer coefficient
            
            % The alpha value computed here will get multiplied with the total cell
            % surface in the simulation model --> We must scale the heat transfer
            % coefficient to the total cell surface.

            % Example for a cell that is cooled from both x-sides and from one y-side:
            % alpha_total = (alpha_x1*A_x + alpha_x2*A_x + alpha_y*A_y) / A_cell
            
            alpha_cell_ambient_vec(ii) = sum(alpha_channel(row) .* A_heat_total_cell) / A_cell_total;
        
        end
end
end
